simulink subsystem "Brytarsystem_Precharge"  (R2020b)
settings: Solver=VariableStepAuto  StartTime=0.0  StopTime=10.0  RelTol=1e-3
libraries: ee_lib x15, fl_lib x7, nesl_utility x3, eeGeneralControl x1
settings Model: Creator=David  LastModifiedBy=David

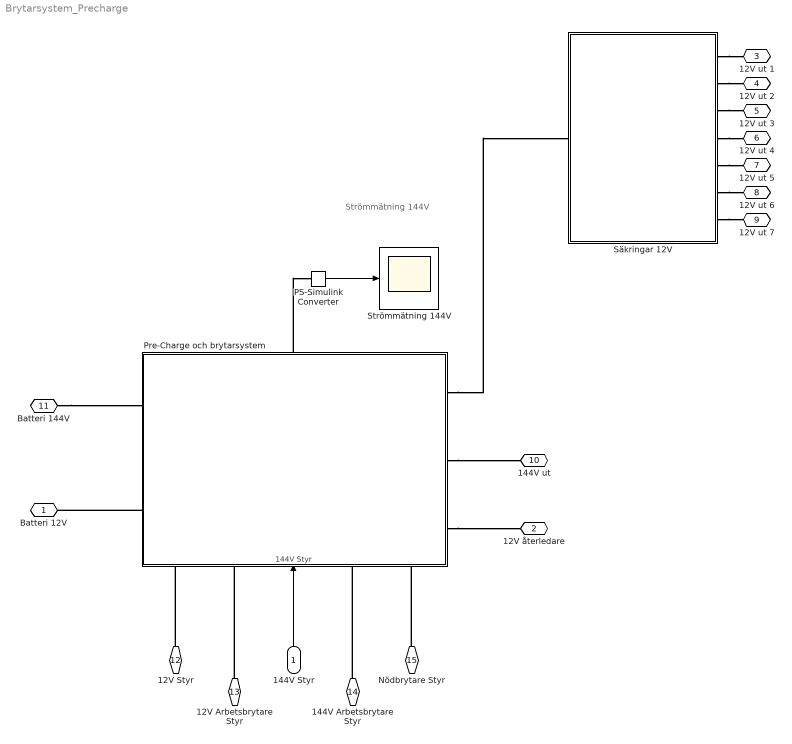
== system Brytarsystem_Precharge ==
  note: Strömmätning 144V
  144V Styr : Inport
  PS-Simulink Converter : nesl_utility/PS-Simulink Converter  PhysicalDomain=network_engine_domain  SubClassName=ps_output  LeftPortType=input  RightPortType=output  PseudoPeriodic=off  Frequencies=[]  Unit=inherit  AffineConversion=off
  Pre-Charge och brytarsystem : Subsystem
      settings: PortSchema="{\"entries\":[{\"content\":{\"sides\":[{\"content\":{\"connectorIds\":[\"LConn1\",\"LConn2\"]},\"type\":\"ConnectorPlacement.EquallySpacedRectSide\",\"uuid\":\"290361da-6fff-44cf-bb1e-6bbb0be8b53d\"},{\"content\":{\"connectorIds\":[\"RConn1\",\"RConn2\",\"RConn3\"],\"side\":\"RIGHT\"},\"type\":\"ConnectorPlacement.EquallySpacedRectSide\",\"uuid\":\"dfbebf99-0128-45e3-b562-be8164f33261\"},{\"content\":{\"connectorIds\":[\"LConn3\"],\"side\":\"TOP\"},\"type\":\"ConnectorPlacement.EquallySpacedRectSide\",\"uuid\":\"6c83dbed-513d-4278-afa8-1a48fd8db2d3\"},{\"content\":{\"connectorIds\":[\"RConn4\",\"RConn5\",\"In1\",\"RConn6\",\"RConn7\"],\"side\":\"BOTTOM\"},\"type\":\"ConnectorPlacement.EquallySpacedRectSide\",\"uuid\":\"403c0301-c3b3-4654-b126-08785e78ac91\"},{\"content\":{\"connectorIds\":[],\"side\":\"HIDDEN\"},\"type\":\"ConnectorPlacement.EquallySpacedRectSide\",\"uuid\":\"4afc1228-53cb-4fb6-bc76-179ada99e2d2\"}]},\"type\":\"ConnectorPlacement.EquallySpacedConnector\",\"uuid\":\"6b1f2643-d83f-4ec7-852e-4ed199232a75\"}],\"packageUris\":[\"http://schema.mathworks.com/mf0/Connector/R2020b\"],\"version\":\"1.0\"}"
  Strömmätning 144V : Scope
  Säkringar 12V : Subsystem
  Batteri 12V : PMIOPort  Side=Left
  "12V återledare " : PMIOPort  Port=2  Side=Left
  12V ut 1 : PMIOPort  Port=3  Side=Right
  12V ut 2 : PMIOPort  Port=4  Side=Right
  12V ut 3 : PMIOPort  Port=5  Side=Right
  12V ut 4 : PMIOPort  Port=6  Side=Right
  12V ut 5 : PMIOPort  Port=7  Side=Right
  12V ut 6 : PMIOPort  Port=8  Side=Right
  12V ut 7 : PMIOPort  Port=9  Side=Right
  144V ut : PMIOPort  Port=10  Side=Right
  Batteri 144V : PMIOPort  Port=11  Side=Left
  12V Styr : PMIOPort  Port=12  Side=Left
  12V Arbetsbrytare Styr : PMIOPort  Port=13  Side=Left
  144V Arbetsbrytare Styr : PMIOPort  Port=14  Side=Left
  Nödbrytare Styr : PMIOPort  Port=15  Side=Left
  wires:
  PS-Simulink Converter/1 -> Strömmätning 144V/1
  144V Styr/1 -> Pre-Charge och brytarsystem/1(144V Styr)
  connections:
  Batteri 144V/RConn1 -- Pre-Charge och brytarsystem/LConn1
  Säkringar 12V/RConn2 -- 12V ut 2/RConn1
  Pre-Charge och brytarsystem/LConn2 -- Batteri 12V/RConn1
  Pre-Charge och brytarsystem/RConn3 -- "12V återledare "/RConn1
  Pre-Charge och brytarsystem/LConn3 -- PS-Simulink Converter/LConn1
  Pre-Charge och brytarsystem/RConn2 -- 144V ut/RConn1
  Pre-Charge och brytarsystem/RConn1 -- Säkringar 12V/LConn1
  Säkringar 12V/RConn1 -- 12V ut 1/RConn1
  Säkringar 12V/RConn3 -- 12V ut 3/RConn1
  Säkringar 12V/RConn5 -- 12V ut 5/RConn1
  Säkringar 12V/RConn4 -- 12V ut 4/RConn1
  Säkringar 12V/RConn7 -- 12V ut 7/RConn1
  Säkringar 12V/RConn6 -- 12V ut 6/RConn1
  12V Styr/RConn1 -- Pre-Charge och brytarsystem/RConn4
  12V Arbetsbrytare Styr/RConn1 -- Pre-Charge och brytarsystem/RConn5
  144V Arbetsbrytare Styr/RConn1 -- Pre-Charge och brytarsystem/RConn6
  Nödbrytare Styr/RConn1 -- Pre-Charge och brytarsystem/RConn7

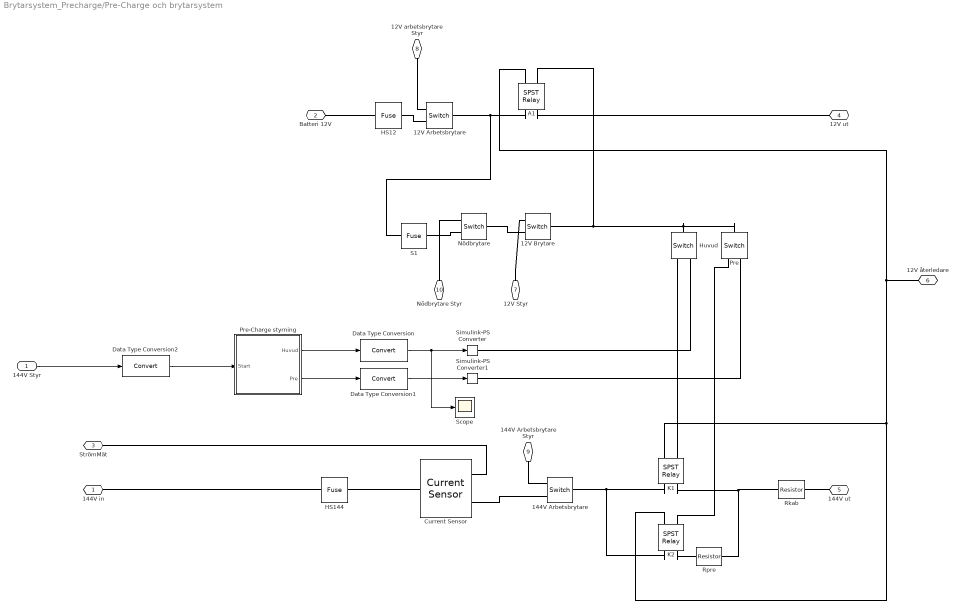
== system Brytarsystem_Precharge/Pre-Charge och brytarsystem ==
  144V Styr : Inport
  12V Arbetsbrytare : fl_lib/Electrical/Electrical Elements/Switch  R_closed=0.01 Ohm  G_open=1e-8 1/Ohm  Threshold=0.5  i_specify=off  i_priority=None  i=0 A  i_nominal_specify=off  i_nominal_unit=A  i_nominal_value=1  v_specify=off  v_priority=None  v=0 V  v_nominal_specify=off  v_nominal_unit=V  v_nominal_value=1
  "12V Brytare " : fl_lib/Electrical/Electrical Elements/Switch  R_closed=0.01 Ohm  G_open=1e-8 1/Ohm  Threshold=0.5  i_specify=off  i_priority=None  i=0 A  i_nominal_specify=off  i_nominal_unit=A  i_nominal_value=1  v_specify=off  v_priority=None  v=0 V  v_nominal_specify=off  v_nominal_unit=V  v_nominal_value=1
  144V Arbetsbrytare : fl_lib/Electrical/Electrical Elements/Switch  R_closed=0.01 Ohm  G_open=1e-8 1/Ohm  Threshold=0.5  i_specify=off  i_priority=None  i=0 A  i_nominal_specify=off  i_nominal_unit=A  i_nominal_value=1  v_specify=off  v_priority=None  v=0 V  v_nominal_specify=off  v_nominal_unit=V  v_nominal_value=1
  A1 : ee_lib/Switches & Breakers/Relays/SPST Relay  block_choices=ee.enum.controlport.elec  R_closed=0.01 Ohm  G_open=1e-8 1/Ohm  Threshold=0  exposemeasurement=ee.enum.exposemeasurement.hidden  T_brk_C_S=0 s  T_mak_C_S=0 s  V_rated=12 V  V_energize=75  V_deenergize=25  l_winding=0.08 H  r_winding=2400 Ohm  g_winding=1e-9 1/Ohm  enable_faults=ee.enum.relays.enable.no  fault_action=ee.enum.relays.faultaction.none  fault_types=ee.enum.relays.faultTypes.winding  fault_condition_ps=ee.enum.relays.faultConditionSPSTps.csstuck  r_deg_closed_s=1e-9 Ohm  winding_tau_fault=1e-3 s  tau_fault=1e-3 s  enable_temporal_fault=ee.enum.relays.enable.no  t_fault_stick=1 s  t_fault_ComOpen=1 s  t_fault=1 s  enable_behavioral_fault=ee.enum.relays.enable.no  winding_max_permissible_voltage=inf V  n_fail_on_voltage=1  winding_max_permissible_current=inf A  max_permissible_current=inf A  t_fail_on_current=1 s
      settings: SourceProductBaseCode=PS  InternalSimscapePortConfiguration="{\"Bottom\":[],\"Left\":[{\"id\":\"p_winding\",\"label\":\"+\",\"type\":\"foundation.electrical.electrical\"},{\"id\":\"n_winding\",\"label\":\"-\",\"type\":\"foundation.electrical.electrical\"}],\"Right\":[{\"id\":\"S\",\"label\":\"S\",\"type\":\"foundation.electrical.electrical\"},{\"id\":\"COM\",\"label\":\"C\",\"type\":\"foundation.electrical.electrical\"}],\"Top\":[]}"
  Current Sensor : fl_lib/Electrical/Electrical Sensors/Current Sensor
  Data Type Conversion : DataTypeConversion
  Data Type Conversion1 : DataTypeConversion
  Data Type Conversion2 : DataTypeConversion
  HS12 : ee_lib/Switches & Breakers/Fuse  prm=1  I_rated=16 A  melt_margin=1  T_fuse=0 s  I2t=1 s*A^2  I_vec=[1.9, 2, 2.5, 30] A  t_vec=[10000, 1, .3, .001] s  R_closed=0.01 Ohm  G_open=1e-8 1/Ohm  exposemeasurement=ee.enum.exposemeasurement.hidden
      settings: SourceProductBaseCode=PS  InternalSimscapePortConfiguration="{\"Bottom\":[],\"Left\":[{\"id\":\"p\",\"label\":\"\",\"type\":\"foundation.electrical.electrical\"}],\"Right\":[{\"id\":\"n\",\"label\":\"\",\"type\":\"foundation.electrical.electrical\"}],\"Top\":[]}"
  HS144 : ee_lib/Switches & Breakers/Fuse  prm=1  I_rated=250 A  melt_margin=1  T_fuse=0 s  I2t=1 s*A^2  I_vec=[1.9, 2, 2.5, 30] A  t_vec=[10000, 1, .3, .001] s  R_closed=0.01 Ohm  G_open=1e-8 1/Ohm  exposemeasurement=ee.enum.exposemeasurement.hidden
      settings: SourceProductBaseCode=PS  InternalSimscapePortConfiguration="{\"Bottom\":[],\"Left\":[{\"id\":\"p\",\"label\":\"\",\"type\":\"foundation.electrical.electrical\"}],\"Right\":[{\"id\":\"n\",\"label\":\"\",\"type\":\"foundation.electrical.electrical\"}],\"Top\":[]}"
  Huvud : fl_lib/Electrical/Electrical Elements/Switch  R_closed=0.01 Ohm  G_open=1e-8 1/Ohm  Threshold=0.5  i_specify=off  i_priority=None  i=0 A  i_nominal_specify=off  i_nominal_unit=A  i_nominal_value=1  v_specify=off  v_priority=None  v=0 V  v_nominal_specify=off  v_nominal_unit=V  v_nominal_value=1
      settings: LogSimulationData=on
  K1 : ee_lib/Switches & Breakers/Relays/SPST Relay  block_choices=ee.enum.controlport.elec  R_closed=0.01 Ohm  G_open=1e-8 1/Ohm  Threshold=0  exposemeasurement=ee.enum.exposemeasurement.hidden  T_brk_C_S=0 s  T_mak_C_S=0 s  V_rated=12 V  V_energize=75  V_deenergize=25  l_winding=0.08 H  r_winding=1700 Ohm  g_winding=1e-9 1/Ohm  enable_faults=ee.enum.relays.enable.no  fault_action=ee.enum.relays.faultaction.none  fault_types=ee.enum.relays.faultTypes.winding  fault_condition_ps=ee.enum.relays.faultConditionSPSTps.csstuck  r_deg_closed_s=1e-9 Ohm  winding_tau_fault=1e-3 s  tau_fault=1e-3 s  enable_temporal_fault=ee.enum.relays.enable.no  t_fault_stick=1 s  t_fault_ComOpen=1 s  t_fault=1 s  enable_behavioral_fault=ee.enum.relays.enable.no  winding_max_permissible_voltage=inf V  n_fail_on_voltage=1  winding_max_permissible_current=inf A  max_permissible_current=inf A  t_fail_on_current=1 s
      settings: SourceProductBaseCode=PS  InternalSimscapePortConfiguration="{\"Bottom\":[],\"Left\":[{\"id\":\"p_winding\",\"label\":\"+\",\"type\":\"foundation.electrical.electrical\"},{\"id\":\"n_winding\",\"label\":\"-\",\"type\":\"foundation.electrical.electrical\"}],\"Right\":[{\"id\":\"S\",\"label\":\"S\",\"type\":\"foundation.electrical.electrical\"},{\"id\":\"COM\",\"label\":\"C\",\"type\":\"foundation.electrical.electrical\"}],\"Top\":[]}"
  K2 : ee_lib/Switches & Breakers/Relays/SPST Relay  block_choices=ee.enum.controlport.elec  R_closed=0.01 Ohm  G_open=1e-8 1/Ohm  Threshold=0  exposemeasurement=ee.enum.exposemeasurement.hidden  T_brk_C_S=0 s  T_mak_C_S=0 s  V_rated=12 V  V_energize=75  V_deenergize=25  l_winding=0.08 H  r_winding=1700 Ohm  g_winding=1e-9 1/Ohm  enable_faults=ee.enum.relays.enable.no  fault_action=ee.enum.relays.faultaction.none  fault_types=ee.enum.relays.faultTypes.winding  fault_condition_ps=ee.enum.relays.faultConditionSPSTps.csstuck  r_deg_closed_s=1e-9 Ohm  winding_tau_fault=1e-3 s  tau_fault=1e-3 s  enable_temporal_fault=ee.enum.relays.enable.no  t_fault_stick=1 s  t_fault_ComOpen=1 s  t_fault=1 s  enable_behavioral_fault=ee.enum.relays.enable.no  winding_max_permissible_voltage=inf V  n_fail_on_voltage=1  winding_max_permissible_current=inf A  max_permissible_current=inf A  t_fail_on_current=1 s
      settings: SourceProductBaseCode=PS  InternalSimscapePortConfiguration="{\"Bottom\":[],\"Left\":[{\"id\":\"p_winding\",\"label\":\"+\",\"type\":\"foundation.electrical.electrical\"},{\"id\":\"n_winding\",\"label\":\"-\",\"type\":\"foundation.electrical.electrical\"}],\"Right\":[{\"id\":\"S\",\"label\":\"S\",\"type\":\"foundation.electrical.electrical\"},{\"id\":\"COM\",\"label\":\"C\",\"type\":\"foundation.electrical.electrical\"}],\"Top\":[]}"
  Nödbrytare : fl_lib/Electrical/Electrical Elements/Switch  R_closed=0.01 Ohm  G_open=1e-8 1/Ohm  Threshold=0.5  i_specify=off  i_priority=None  i=0 A  i_nominal_specify=off  i_nominal_unit=A  i_nominal_value=1  v_specify=off  v_priority=None  v=0 V  v_nominal_specify=off  v_nominal_unit=V  v_nominal_value=1
  Pre : fl_lib/Electrical/Electrical Elements/Switch  R_closed=0.01 Ohm  G_open=1e-8 1/Ohm  Threshold=0.5  i_specify=off  i_priority=None  i=0 A  i_nominal_specify=off  i_nominal_unit=A  i_nominal_value=1  v_specify=off  v_priority=None  v=0 V  v_nominal_specify=off  v_nominal_unit=V  v_nominal_value=1
      settings: LogSimulationData=on
  Pre-Charge styrning : Subsystem
  Rkab : ee_lib/Passive/Resistor  R=1.1e-5 Ohm  R_tol=5  enable_R_tol=0  tol_distribution=1  nSigma=4  enable_operating_limits=0  operating_limit_action=2  max_working_voltage=100 V  power_rating=1 W  enable_faults=0  fault_action=1  R_faulted=inf Ohm  enable_temporal_fault=0  t_fault=1 s  enable_behavioral_fault=0  max_permissible_current=1 A  t_fail_on_current=1 s  noise_mode=0  sample_time=1e-3 s  repeatability=1  auto_seed=1125905567  user_seed=0  Tdevice=25 degC  alpha=3.93e-3 1/K  Tmeas=25 degC  thermal_mass=100 J/K  power_derating_T1=70 degC  power_derating_T2=155 degC  operating_temperature_range_vec=[-50, 150] degC  temperature_specify=off  temperature_priority=High  temperature=298.15 K  temperature_nominal_specify=off  temperature_nominal_unit=K  temperature_nominal_value=1
      settings: LogSimulationData=on
  Rpre : ee_lib/Passive/Resistor  R=0.75 Ohm  R_tol=5  enable_R_tol=0  tol_distribution=1  nSigma=4  enable_operating_limits=0  operating_limit_action=2  max_working_voltage=100 V  power_rating=1 W  enable_faults=0  fault_action=1  R_faulted=inf Ohm  enable_temporal_fault=0  t_fault=1 s  enable_behavioral_fault=0  max_permissible_current=1 A  t_fail_on_current=1 s  noise_mode=0  sample_time=1e-3 s  repeatability=1  auto_seed=190928873  user_seed=0  Tdevice=25 degC  alpha=3.93e-3 1/K  Tmeas=25 degC  thermal_mass=100 J/K  power_derating_T1=70 degC  power_derating_T2=155 degC  operating_temperature_range_vec=[-50, 150] degC  temperature_specify=off  temperature_priority=High  temperature=298.15 K  temperature_nominal_specify=off  temperature_nominal_unit=K  temperature_nominal_value=1
      settings: LogSimulationData=on
  S1 : ee_lib/Switches & Breakers/Fuse  prm=1  I_rated=10 A  melt_margin=1  T_fuse=0 s  I2t=1 s*A^2  I_vec=[1.9, 2, 2.5, 30] A  t_vec=[10000, 1, .3, .001] s  R_closed=0.01 Ohm  G_open=1e-8 1/Ohm  exposemeasurement=ee.enum.exposemeasurement.hidden
      settings: SourceProductBaseCode=PS  InternalSimscapePortConfiguration="{\"Bottom\":[],\"Left\":[{\"id\":\"p\",\"label\":\"\",\"type\":\"foundation.electrical.electrical\"}],\"Right\":[{\"id\":\"n\",\"label\":\"\",\"type\":\"foundation.electrical.electrical\"}],\"Top\":[]}"
  Scope : Scope
  Simulink-PS Converter : nesl_utility/Simulink-PS Converter  PhysicalDomain=network_engine_domain  SubClassName=ps_input  LeftPortType=input  RightPortType=output  PseudoPeriodic=off  Frequencies=[]  NoiseDistribution=none  NoiseParameters=[]  Unit=1  AffineConversion=off  FilteringAndDerivatives=provide  SimscapeFilterOrder=1  InputFilterTimeConstant=0.001  UdotUserProvided=0
  Simulink-PS Converter1 : nesl_utility/Simulink-PS Converter  PhysicalDomain=network_engine_domain  SubClassName=ps_input  LeftPortType=input  RightPortType=output  PseudoPeriodic=off  Frequencies=[]  NoiseDistribution=none  NoiseParameters=[]  Unit=1  AffineConversion=off  FilteringAndDerivatives=provide  SimscapeFilterOrder=1  InputFilterTimeConstant=0.001  UdotUserProvided=0
  144V in : PMIOPort  Side=Left
  Batteri 12V : PMIOPort  Port=2  Side=Left
  StrömMät : PMIOPort  Port=3  Side=Left
  12V ut : PMIOPort  Port=4  Side=Right
  144V ut : PMIOPort  Port=5  Side=Right
  "12V återledare " : PMIOPort  Port=6  Side=Right
  12V Styr : PMIOPort  Port=7  Side=Right
  12V arbetsbrytare Styr : PMIOPort  Port=8  Side=Right
  144V Arbetsbrytare Styr : PMIOPort  Port=9  Side=Right
  Nödbrytare Styr : PMIOPort  Port=10  Side=Right
  wires:
  Data Type Conversion/1 -> Scope/1, Simulink-PS Converter/1
  Data Type Conversion1/1 -> Simulink-PS Converter1/1
  Pre-Charge styrning/2(Pre) -> Data Type Conversion1/1
  Pre-Charge styrning/1(Huvud) -> Data Type Conversion/1
  Data Type Conversion2/1 -> Pre-Charge styrning/1(Start)
  144V Styr/1 -> Data Type Conversion2/1
  connections:
  A1/RConn1 -- 12V ut/RConn1
  Simulink-PS Converter/RConn1 -- Huvud/RConn1
  144V Arbetsbrytare/RConn2 -- Current Sensor/RConn2
  Nödbrytare/LConn1 -- "12V Brytare "/RConn2
  Current Sensor/LConn1 -- HS144/RConn1
  Huvud/RConn2 -- K1/LConn1
  Pre/RConn2 -- K2/LConn1
  Simulink-PS Converter1/RConn1 -- Pre/RConn1
  Current Sensor/RConn1 -- StrömMät/RConn1
  K2/RConn1 -- Rpre/LConn1
  K2/RConn2 -- 144V Arbetsbrytare/LConn1 -- K1/RConn2
  Nödbrytare/RConn2 -- S1/RConn1
  A1/RConn2 -- 12V Arbetsbrytare/LConn1 -- S1/LConn1
  Nödbrytare Styr/RConn1 -- Nödbrytare/RConn1
  144V Arbetsbrytare Styr/RConn1 -- 144V Arbetsbrytare/RConn1
  A1/LConn1 -- Pre/LConn1 -- Huvud/LConn1 -- "12V Brytare "/LConn1
  12V Arbetsbrytare/RConn2 -- HS12/RConn1
  12V Arbetsbrytare/RConn1 -- 12V arbetsbrytare Styr/RConn1
  A1/LConn2 -- K1/LConn2 -- K2/LConn2 -- "12V återledare "/RConn1
  12V Styr/RConn1 -- "12V Brytare "/RConn1
  144V in/RConn1 -- HS144/LConn1
  K1/RConn1 -- Rkab/LConn1 -- Rpre/RConn1
  Batteri 12V/RConn1 -- HS12/LConn1
  144V ut/RConn1 -- Rkab/RConn1

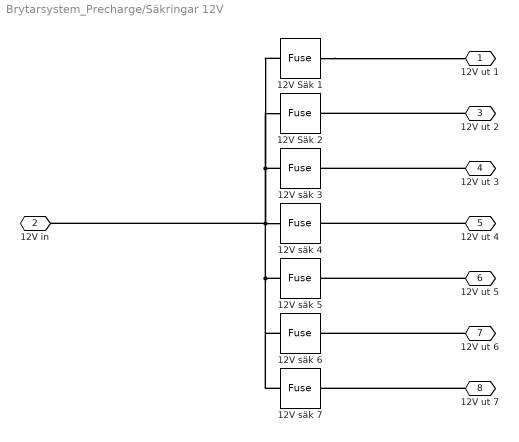
== system Brytarsystem_Precharge/Säkringar 12V ==
  12V Säk 1 : ee_lib/Switches & Breakers/Fuse  prm=1  I_rated=10 A  melt_margin=1  T_fuse=0 s  I2t=1 s*A^2  I_vec=[1.9, 2, 2.5, 30] A  t_vec=[10000, 1, .3, .001] s  R_closed=0.01 Ohm  G_open=1e-8 1/Ohm  exposemeasurement=ee.enum.exposemeasurement.hidden
      settings: SourceProductBaseCode=PS  InternalSimscapePortConfiguration="{\"Bottom\":[],\"Left\":[{\"id\":\"p\",\"label\":\"\",\"type\":\"foundation.electrical.electrical\"}],\"Right\":[{\"id\":\"n\",\"label\":\"\",\"type\":\"foundation.electrical.electrical\"}],\"Top\":[]}"
  12V Säk 2 : ee_lib/Switches & Breakers/Fuse  prm=1  I_rated=10 A  melt_margin=1  T_fuse=0 s  I2t=1 s*A^2  I_vec=[1.9, 2, 2.5, 30] A  t_vec=[10000, 1, .3, .001] s  R_closed=0.01 Ohm  G_open=1e-8 1/Ohm  exposemeasurement=ee.enum.exposemeasurement.hidden
      settings: SourceProductBaseCode=PS  InternalSimscapePortConfiguration="{\"Bottom\":[],\"Left\":[{\"id\":\"p\",\"label\":\"\",\"type\":\"foundation.electrical.electrical\"}],\"Right\":[{\"id\":\"n\",\"label\":\"\",\"type\":\"foundation.electrical.electrical\"}],\"Top\":[]}"
  12V säk {3..7} (5 alike) : ee_lib/Switches & Breakers/Fuse  prm=1  I_rated=10 A  melt_margin=1  T_fuse=0 s  I2t=1 s*A^2  I_vec=[1.9, 2, 2.5, 30] A  t_vec=[10000, 1, .3, .001] s  R_closed=0.01 Ohm  G_open=1e-8 1/Ohm  exposemeasurement=ee.enum.exposemeasurement.hidden
      settings: SourceProductBaseCode=PS  InternalSimscapePortConfiguration="{\"Bottom\":[],\"Left\":[{\"id\":\"p\",\"label\":\"\",\"type\":\"foundation.electrical.electrical\"}],\"Right\":[{\"id\":\"n\",\"label\":\"\",\"type\":\"foundation.electrical.electrical\"}],\"Top\":[]}"
  12V ut 1 : PMIOPort  Side=Right
  12V in : PMIOPort  Port=2  Side=Left
  12V ut 2 : PMIOPort  Port=3  Side=Right
  12V ut 3 : PMIOPort  Port=4  Side=Right
  12V ut 4 : PMIOPort  Port=5  Side=Right
  12V ut 5 : PMIOPort  Port=6  Side=Right
  12V ut 6 : PMIOPort  Port=7  Side=Right
  12V ut 7 : PMIOPort  Port=8  Side=Right
  connections:
  12V ut 7/RConn1 -- 12V säk 7/RConn1
  12V ut 6/RConn1 -- 12V säk 6/RConn1
  12V ut 5/RConn1 -- 12V säk 5/RConn1
  12V ut 4/RConn1 -- 12V säk 4/RConn1
  12V Säk 1/RConn1 -- 12V ut 1/RConn1
  12V säk 3/LConn1 -- 12V Säk 2/LConn1 -- 12V Säk 1/LConn1 -- 12V säk 4/LConn1 -- 12V säk 5/LConn1 -- 12V säk 6/LConn1 -- 12V säk 7/LConn1 -- 12V in/RConn1
  12V ut 3/RConn1 -- 12V säk 3/RConn1
  12V ut 2/RConn1 -- 12V Säk 2/RConn1

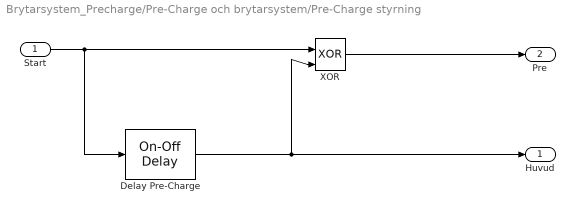
== system Brytarsystem_Precharge/Pre-Charge och brytarsystem/Pre-Charge styrning ==
  Start : Inport
  Delay Pre-Charge : eeGeneralControl/On-Off Delay  LabelModeActiveChoice=Discrete  Td_on=0.05  Td_off=0  IC=0  Ts=0.0001
      settings: SourceProductBaseCode=PS
  XOR : Logic  Operator=XOR  IconShape=distinctive  AllPortsSameDT=off  OutDataTypeStr=boolean
  Huvud : Outport
  Pre : Outport  Port=2
  wires:
  Delay Pre-Charge/1 -> XOR/2, Huvud/1
  Start/1 -> XOR/1, Delay Pre-Charge/1
  XOR/1 -> Pre/1
